simulink model "modelo_serial_red_Neuronal"  (R2019a)
settings: Solver=FixedStepAuto  StartTime=0.0  StopTime=inf  RelTol=1e-3  EnableMultiTasking=on
undefined symbols (not defined in the file): serial
libraries: instrumentlib x3, simulink x3, neural x1
settings Model: ExtModeTrigDuration=2  Creator=Kike  LastModifiedBy=Kike
settings SolverCC: AutoInsertRateTranBlk=on
settings OptimizationCC: EnhancedBackFolding=on  PassReuseOutputArgsAs=Individual arguments  MaxStackSize=64  OptimizeBlockOrder=speed  DifferentSizesBufferReuse=on
settings DebuggingCC: ParameterTunabilityLossMsg=error
settings HardwareCC: ProdBitPerInt=16  ProdBitPerPointer=16  ProdBitPerSizeT=16  ProdBitPerPtrDiffT=16  ProdLargestAtomicFloat=None  ProdWordSize=8  ProdHWDeviceType=Atmel->AVR
settings SFSimCC: MATLABDynamicMemAlloc=off
settings RTWCC: SystemTargetFile=ert.tlc  HardwareBoard=Arduino Nano 3.0  TLCOptions=-aInlineSetEventsForThisBaseRateFcn=TLC_FALSE -aSuppressMultiTaskScheduler=TLC_FALSE -aRateBasedStepFcn=1  TemplateMakefile=ert_default_tmf  GenerateReport=on  Toolchain=Arduino AVR  BuildConfiguration=Faster Runs  IncludeHyperlinkInReport=on  LaunchReport=on  GenerateTraceInfo=on  GenerateTraceReport=on  GenerateTraceReportSl=on  GenerateTraceReportSf=on  GenerateTraceReportEml=on
settings CodeAppCC: ForceParamTrailComments=on  IgnoreCustomStorageClasses=off  OperatorAnnotations=on  SimulinkDataObjDesc=on  SFDataObjDesc=on  InsertBlockDesc=on
settings ERTTargetCC: SupportContinuousTime=on  SupportVariableSizeSignals=on  ExtModeStaticAllocSize=250

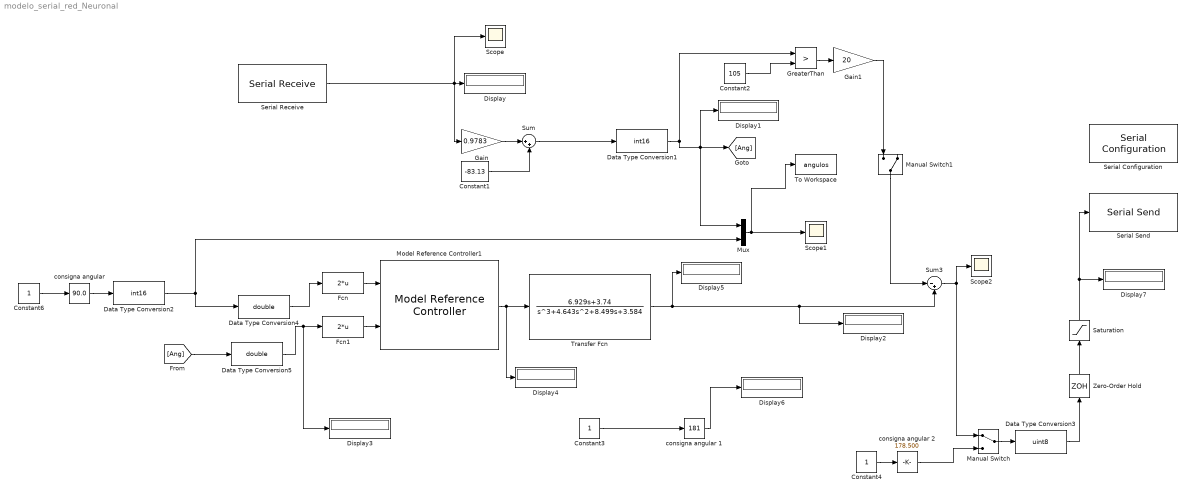
== system modelo_serial_red_Neuronal ==
  Constant1 : Constant  Value=-83.13
  Constant2 : Constant  Value=105  OutDataTypeStr=int16
  Constant3 : Constant
  Constant4 : Constant
  Constant6 : Constant
  Data Type Conversion1 : DataTypeConversion  OutDataTypeStr=int16
  Data Type Conversion2 : DataTypeConversion  OutDataTypeStr=int16
  Data Type Conversion3 : DataTypeConversion  OutDataTypeStr=uint8
  Data Type Conversion4 : DataTypeConversion  OutDataTypeStr=double
  Data Type Conversion5 : DataTypeConversion  OutDataTypeStr=double
  Display{,1..7} (8 alike) : Display
  Fcn : Fcn  Expr=2*u
  Fcn1 : Fcn  Expr=2*u
  Gain : Gain  Gain=0.9783
  Gain1 : Gain  Gain=20
  GreaterThan : RelationalOperator  Operator=>  OutDataTypeStr=boolean  RndMeth=Simplest
  Manual Switch : ManualSwitch
  Manual Switch1 : ManualSwitch  CurrentSetting=0
  Model Reference Controller1 : neural/Control Systems/Model Reference Controller  Nrc=2  Nic=1  Njc=2  IW_y=[-0.044211859364690707375 -0.48109163842484958806;0.24746719845010403671 -0.2782369371412904413;5.3862614114807767507 6.6342903536528243791;-10.776031369529354365 -8.6202595663960472905;-0.71410071005093345153 -0.094595609222146825878;8.0458633184976662278 -8.1880849294468678323;-0.10774689352302514733 -1.8677683713788850728;5.0940912788230647834 3.7309209687155280299;0.016784015788765722227 -0.49092966700431439619;-4.8092055208385469101 2.5291456849304148058;-0.99013933865810677126 0.17471158968958913627;-0.072385764677869890438 0.56153063425737514969;-0.86746726172537413913 -1.3251187272271340856]  IW_u=[-0.63095693721071077764;-0.012729543593183323055;-7.5285741832068397983;-4.3094658530044460676;-1.2167654952042519234;0.0061433550011621282025;-1.389251770970561406;1.1519796724585946723;0.98151008409794959775;3.7881829369347168601;2.0448287302966616785;-0.24415522820949894789;-2.5071554459997567044]  IW_r=[0.43130773072925160383 2.2065521749536265439;-0.74331155311484820025 -0.12204610452285462319;-1.1488874942413276337 0.84673913282715140838;-0.88726397783592336754 3.0024799501343086838;0.97779293775656050958 -1.1910474080130910579;-2.2851382880541692977 -9.60406580112701036;-2.266578072341822736 -1.2447321470757772843;-1.0960677307877235709 -2.2304026288509666287;1.4005273978733330242 -1.2248812534636244198;-10.442669592690423386 -10.368212373738652232;-1.276342332974564453 0.73835231448270677301;2.1170857763530053219 1.3871300566614697125;-1.0256535700547853018 1.5135829498826041117]  B1_c=[2.5527160935935935271;-1.8571547465152644651;-2.4815195860298286945;-1.2591870737811814429;0.38910101958534859534;-4.789015237281883941;4.5504747143580237534;2.0695771161438463182;0.79741252128976736202;6.9677874988703543124;-2.1380336603589240596;-2.1777870203411482386;2.371587991635047743]  B2_c=2.3761177423931871822  LW_c=[0.82216376206536900817 -2.1689608416235461874 -9.425203305454751046 1.9075510542470823783 4.1933692963579654034 4.2252947333561463594 -2.2632775063015460049 -1.1332082707048700687 3.6202660954798302484 -9.9662595704343086567 -2.6260733924236951964 -2.8586814942993306055 7.8572617924047065685]  retraining_c=30  max_i_int=2  min_i_int=0.1  max_r_int=2  min_r_int=0.1  Ts=0.05  S1=10  Ni=2  Nj=2  sim_file=robotref  trainfun=trainlm  Use_validation=1  Use_Testing=1  Use_Inc_training=0  Use_previous_weights=1  max_i=180  min_i=0  max_r=180  min_r=0  sam_training=10000  sam_training_c=6000  epochs=300  epochs_c=10  minp=0.37061195833007598566  maxp=179.29526658282324547  mint=-2.0275241129659207218  maxt=179.29526658282324547  Normalize=1  IW=[0.67556972283606331331 -0.69678512246161106169;-0.0020527679858192253437 -0.0061584526783613861844;0.002741311193177919589 0.0026388182399964565418;-0.0066339439415476963643 -0.0050233266673244602804;0.83882332912818102777 -0.26788237355390781547;-0.0022422785895424872035 -0.0049720434535305470941;-0.40310582519648363586 0.41939516972539536699;-0.57832168978973408358 0.57964213405289022329;-0.0025473313782971695324 -0.0022961362570170593816;-0.0024058355099453453303 -0.0048110562940149896247]  LW1_2=[1.2764115078692681582 -1.3654567742839536226;0.88870418462476896693 1.0009741730127899029;0.32322232485795743262 -0.14841161626950624686;0.71570364781550543931 -0.3623967060322184075;-2.5493375023553004333 -4.1918061837136315617;-0.4868540905107437422 0.13364916593531703248;1.5078988526359184963 -1.780529808989656626;0.58963952392762009058 -0.13785187473585044926;-0.34293254310167370358 0.16518464747230943157;-0.49030311074435617424 0.13318612361388143528]  LW2_1=[0.001794256973857975097 0.0023260266104082895876 4.3375966267596597348 0.38866763861669983982 8.2354560522188442599e-05 2.754895140590533309 0.0092444626355816881397 9.8784717250843917763e-05 -4.4143138817585887423 -2.9220464354292188247]  B1=[8.3454601860294008731;-1.7519137959719046638;0.66842571176574128167;1.9833324392899800426;2.8502821776533338038;-0.0011908754875427425991;-3.0111055895303513452;-1.3200800067551479167;0.88617630901770505503;0.010978045349317493845]  B2=0.26763418406747424561  S1c=13  Limit_output=1  min_output=0  max_output=255  Ref_file=robotref
      settings: SourceProductName=MATLAB Runtime - Deep Learning Toolbox  SourceProductBaseCode=Missing
  Mux : Mux  Inputs=2
  Saturation : Saturate  UpperLimit=255  LowerLimit=0
  Scope : Scope
  Scope1 : Scope
  Scope2 : Scope
  Serial Configuration : instrumentlib/Serial Configuration  Priority=-200000  ComPortMenu=<Please select a port...>  ComPort=COM9  ObjConstructor=serial('COM9');  BaudRate=115200  DataBits=8  Parity=none  StopBits=1  FlowControl=none  Timeout=10  ByteOrder=LittleEndian
  Serial Receive : instrumentlib/Serial Receive  ComPortMenu=<Please select a port...>  ComPort=COM9  ObjConstructor=serial('COM9');  Terminator=<none>  DataSize=1  DataType=uint8  EnableBlockingMode=on  ActionDataUnavailable=Output last received value  CustomValue=0  SampleTime=0.01
  Serial Send : instrumentlib/Serial Send  ComPortMenu=<Please select a port...>  ComPort=COM9  ObjConstructor=serial('COM9');  Terminator=<none>  EnableBlockingMode=on
  Sum : Sum  Inputs=|++
  Sum3 : Sum  Inputs=|-+
  To Workspace : ToWorkspace  VariableName=angulos  SaveFormat=Structure With Time  SampleTime=0.05
  Transfer Fcn : TransferFcn  Numerator=[6.929 3.74]  Denominator=[1 4.643 8.499 3.584]
  Zero-Order Hold : ZeroOrderHold  SampleTime=0.01
  "consigna angular " : simulink/Math Operations/Slider Gain  gain=90.0  low=11.52  high=90
  consigna angular 1 : simulink/Math Operations/Slider Gain  gain=181  low=0  high=255
  consigna angular 2 : simulink/Math Operations/Slider Gain  gain=178.500  low=0  high=255
  wires:
  "consigna angular "/1 -> Data Type Conversion2/1
  Constant1/1 -> Sum/2
  Model Reference Controller1/1 -> Display4/1, Transfer Fcn/1
  Gain/1 -> Sum/1
  Constant3/1 -> consigna angular 1/1
  [Ang] -> Data Type Conversion5/1
  Manual Switch/1 -> Data Type Conversion3/1
  Zero-Order Hold/1 -> Saturation/1
  Constant4/1 -> consigna angular 2/1
  consigna angular 2/1 -> Manual Switch/2
  Mux/1 -> To Workspace/1, Scope1/1
  Saturation/1 -> Serial Send/1, Display7/1
  Serial Receive/1 -> Scope/1, Display/1, Gain/1
  Sum/1 -> Data Type Conversion1/1
  Data Type Conversion1/1 -> Mux/1, [Ang], Display1/1, GreaterThan/1
  Data Type Conversion3/1 -> Zero-Order Hold/1
  Constant2/1 -> GreaterThan/2
  Transfer Fcn/1 -> Display2/1, Sum3/2, Display5/1
  Sum3/1 -> Manual Switch/1, Scope2/1
  GreaterThan/1 -> Gain1/1
  consigna angular 1/1 -> Display6/1
  Constant6/1 -> "consigna angular "/1
  Manual Switch1/1 -> Sum3/1
  Gain1/1 -> Manual Switch1/1
  Data Type Conversion2/1 -> Data Type Conversion4/1, Mux/2
  Data Type Conversion4/1 -> Fcn/1
  Fcn/1 -> Model Reference Controller1/1
  Fcn1/1 -> Model Reference Controller1/2
  Data Type Conversion5/1 -> Display3/1, Fcn1/1
